simulink model "LEO_MPC_SpeedCtrl"  (Simulink 8.2)
settings: Solver=ode45  StartTime=0.0  StopTime=50  RelTol=1e-3
libraries: Solver_SF x1
settings Model: Creator=admin  LastModifiedBy=leoking99
settings DataIOCC: SignalLoggingSaveFormat=Dataset
settings OptimizationCC: ExpressionDepthLimit=128
settings DebuggingCC: FcnCallInpInsideContextMsg=EnableAllAsError  StateNameClashWarn=none
settings GRTTargetCC: CombineOutputUpdateFcns=on  GRTInterface=off

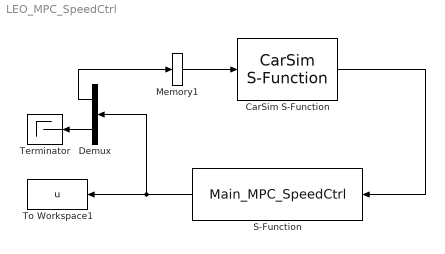
== system LEO_MPC_SpeedCtrl ==
  CarSim S-Function : Solver_SF/CarSim S-Function  Priority=1  VehicleCode=i_i  SIMFILE=LEO_MPC_SpeedCtrl.sim
  Demux : Demux  Outputs=[2 4]
  Memory1 : Memory
  S-Function : S-Function  FunctionName=Main_MPC_SpeedCtrl  EnableBusSupport=off
  Terminator : Terminator
  To Workspace1 : ToWorkspace  VariableName=u  SampleTime=-1  SaveFormat=Structure
  wires:
  S-Function/1 -> Demux/1, To Workspace1/1
  Demux/1 -> Memory1/1
  Demux/2 -> Terminator/1
  CarSim S-Function/1 -> S-Function/1
  Memory1/1 -> CarSim S-Function/1
